simulink model "Lotka_Voltera"  (R2021a)
settings: Solver=ode15s  StartTime=0.0  StopTime=10.0  FixedStep=0.1  RelTol=1e-3  EnableMultiTasking=on
settings Model: Creator=acalame  LastModifiedBy=acalame
settings SolverCC: AlgebraicLoopSolver=TrustRegion  AutoInsertRateTranBlk=on
settings DataIOCC: LimitDataPoints=on
settings OptimizationCC: LifeSpan=inf
settings DebuggingCC: AllowSymbolicDim=off  SFUnexpectedBacktrackingDiag=warning  SFNoUnconditionalDefaultTransitionDiag=warning  SFExecutionAtInitializationDiag=none  ArithmeticOperatorsInVariantConditions=warning
settings SFSimCC: SimUseLocalCustomCode=off  CustomCodeUndefinedFunction=UseInterfaceOnly
settings RTWCC: RTWUseLocalCustomCode=off
settings CodeAppCC: StateflowObjectComments=on
settings GRTTargetCC: TargetLangStandard=C89/C90 (ANSI)
settings ConfigComp: CovMetricSettings=dw  CovSaveCumulativeToWorkspaceVar=on  CovSaveSingleToWorkspaceVar=on  CovExternalEMLEnable=off  CovSFcnEnable=off

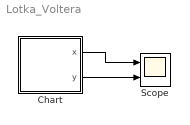
== system Lotka_Voltera ==
  Chart : Stateflow chart  TreatAsAtomicUnit=on
  Scope : Scope  NumInputPorts=2
  wires:
  Chart/1(x) -> Scope/1
  Chart/2(y) -> Scope/2

== stateflow chart Lotka_Voltera/Chart ==
  settings: updateMethod=CONTINUOUS
  state evolution_de_requin_et_sardine
    during :
    x_dot = a*x - b*x*y;
    y_dot =  c*x*y - d*y;
  state evolution_de_requin_et_sardine_peche
    during :
    x_dot = a*x - b*x*y - f*x;
    y_dot =  c*x*y - d*y;
  (default) -> evolution_de_requin_et_sardine : {x=3.33, y = 4}
  evolution_de_requin_et_sardine -> evolution_de_requin_et_sardine_peche : [x>xmax]
  evolution_de_requin_et_sardine_peche -> evolution_de_requin_et_sardine : [x<xmin]
  data: a local =2; b local =1; x output =3.33; y output =4; d local =1; c local =0.3; f local =1; xmax local =3.4; xmin local =3.2
  data x settings: updateMethod=SF_CONTINUOUS_TIME_DATA
  data y settings: updateMethod=SF_CONTINUOUS_TIME_DATA
